simulink model "Controllerlab1"  (R2020a)
settings: Solver=VariableStepAuto  StartTime=0.0  StopTime=10.0  RelTol=1e-3
PostLoadFcn:
  | Kp = 36;
  | Ki = 4;
  | Ts = 0.01;
settings Model: Creator=Anjali123  LastModifiedBy=Anjali123

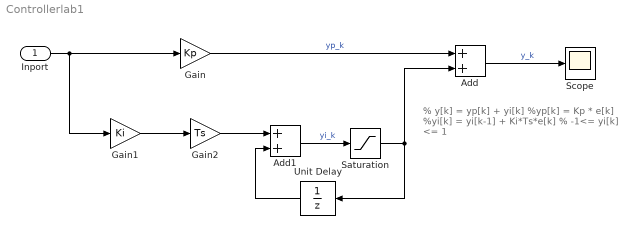
== system Controllerlab1 ==
  note: % y[k] = yp[k] + yi[k]
      | %yp[k] = Kp * e[k]
      | %yi[k] = yi[k-1] + Ki*Ts*e[k]
      | % -1<= yi[k] <= 1
  Inport : Inport
  Add : Sum
  Add1 : Sum
  Gain : Gain  Gain=Kp
  Gain1 : Gain  Gain=Ki
  Gain2 : Gain  Gain=Ts
  Saturation : Saturate  UpperLimit=1  LowerLimit=-1
  Scope : Scope
  Unit Delay : UnitDelay  SampleTime=-1  HasFrameUpgradeWarning=on
  wires:
  Saturation/1 -> Add/2, Unit Delay/1
  Inport/1 -> Gain1/1, Gain/1
  Gain/1 -> Add/1  "yp_k"
  Add/1 -> Scope/1  "y_k"
  Gain1/1 -> Gain2/1
  Gain2/1 -> Add1/1
  Unit Delay/1 -> Add1/2
  Add1/1 -> Saturation/1  "yi_k"
